simulink model "Chess_method_sowing_4_article"  (R2018b)
settings: Solver=FixedStepAuto  StartTime=0.0  StopTime=inf  FixedStep=0.01  MaxStep=0.01  MinStep=0.001  RelTol=1e-3  AbsTol=1e-3  EnableMultiTasking=on
libraries: fl_lib x6, nesl_utility x5, elec_lib x1
settings Model: Creator=Admin  LastModifiedBy=Admin
settings SolverCC: AutoInsertRateTranBlk=on  InsertRTBMode=Always

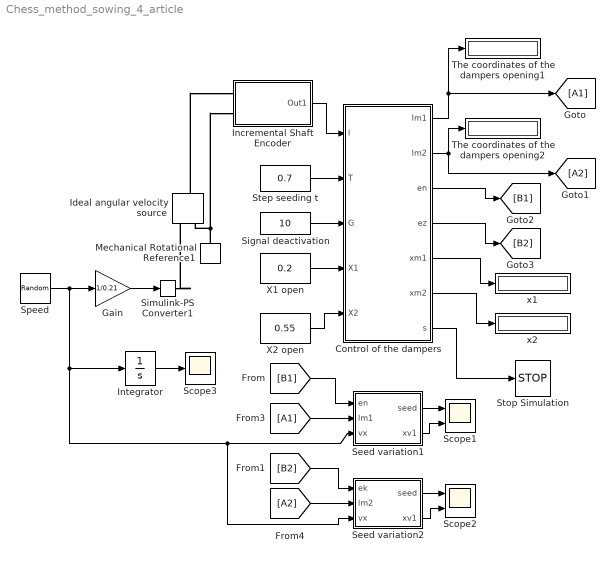
== system Chess_method_sowing_4_article ==
  Control of the dampers : MATLAB Function  TreatAsAtomicUnit=on
  Gain : Gain  Gain=1/0.21
  Ideal angular velocity source : fl_lib/Mechanical/Mechanical Sources/Ideal Angular Velocity Source
  Incremental Shaft Encoder : Subsystem
  Integrator : Integrator
  Mechanical Rotational Reference1 : fl_lib/Mechanical/Rotational Elements/Mechanical Rotational Reference
  Scope1 : Scope  NumInputPorts=2
  Scope2 : Scope  NumInputPorts=2
  Scope3 : Scope
  Seed variation1 : Subsystem
  Seed variation2 : Subsystem
  Signal deactivation : Constant  Value=10
  Simulink-PS Converter1 : nesl_utility/Simulink-PS Converter  PhysicalDomain=network_engine_domain  SubClassName=ps_input  LeftPortType=input  RightPortType=output  PseudoPeriodic=off  Frequencies=[]  NoiseDistribution=none  NoiseParameters=[]  Unit=rad/s  AffineConversion=off  FilteringAndDerivatives=provide  SimscapeFilterOrder=1  InputFilterTimeConstant=0.001  UdotUserProvided=0
  Speed : RandomNumber  Mean=2.5  Variance=0.1  SampleTime=0.1
  Step seeding t : Constant  Value=0.7
  Stop Simulation : Stop
  The coordinates of the dampers opening1 : Display
      settings: Format=bank
  The coordinates of the dampers opening2 : Display
      settings: Format=bank
  X1 open : Constant  Value=0.2  VectorParams1D=off
  X2 open : Constant  Value=0.55  VectorParams1D=off
  x1 : Display
      settings: Format=bank
  x2 : Display
      settings: Format=bank
  wires:
  Step seeding t/1 -> Control of the dampers/2(T)
  Control of the dampers/7(s) -> Stop Simulation/1
  Signal deactivation/1 -> Control of the dampers/3(G)
  X2 open/1 -> Control of the dampers/5(X2)
  Control of the dampers/6(xm2) -> x2/1
  Control of the dampers/5(xm1) -> x1/1
  X1 open/1 -> Control of the dampers/4(X1)
  Seed variation1/1(seed) -> Scope1/1
  Integrator/1 -> Scope3/1
  Speed/1 -> Seed variation1/3(vx), Seed variation2/3(vx), Integrator/1, Gain/1
  Seed variation1/2(xv1) -> Scope1/2
  [A1] -> Seed variation1/2(lm1)
  [A2] -> Seed variation2/2(lm2)
  Seed variation2/1(seed) -> Scope2/1
  Control of the dampers/2(lm2) -> The coordinates of the dampers opening2/1, [A2]
  Control of the dampers/1(lm1) -> [A1], The coordinates of the dampers opening1/1
  Seed variation2/2(xv1) -> Scope2/2
  Control of the dampers/3(en) -> [B1]
  Control of the dampers/4(ez) -> [B2]
  [B1] -> Seed variation1/1(en)
  [B2] -> Seed variation2/1(ek)
  Gain/1 -> Simulink-PS Converter1/1
  Incremental Shaft Encoder/1(Out1) -> Control of the dampers/1(l)
  connections:
  Simulink-PS Converter1/RConn1 -- Ideal angular velocity source/RConn1
  Mechanical Rotational Reference1/LConn1 -- Incremental Shaft Encoder/LConn2 -- Ideal angular velocity source/RConn2
  Ideal angular velocity source/LConn1 -- Incremental Shaft Encoder/LConn1

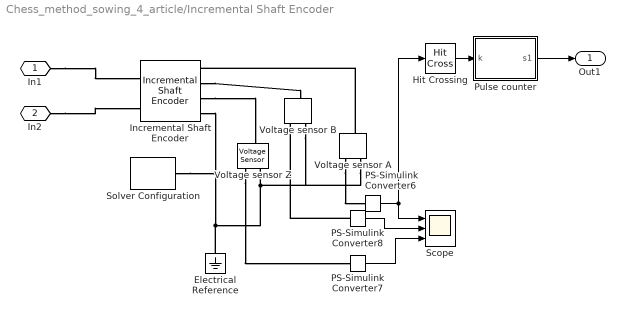
== system Chess_method_sowing_4_article/Incremental Shaft Encoder ==
  Electrical Reference : fl_lib/Electrical/Electrical Elements/Electrical Reference
  Hit Crossing : HitCross  HitCrossingOffset=0.6  HitCrossingDirection=rising
  Incremental Shaft Encoder : elec_lib/Sensors/Incremental Shaft Encoder  NPulse=852  Vm=1 V  angle0=0 rad
      settings: SourceProductName=Simscape Electronics  SourceProductBaseCode=SN
  PS-Simulink Converter6 : nesl_utility/PS-Simulink Converter  PhysicalDomain=network_engine_domain  SubClassName=ps_output  LeftPortType=input  RightPortType=output  PseudoPeriodic=off  Frequencies=[]  Unit=1  AffineConversion=off
  PS-Simulink Converter7 : nesl_utility/PS-Simulink Converter  PhysicalDomain=network_engine_domain  SubClassName=ps_output  LeftPortType=input  RightPortType=output  PseudoPeriodic=off  Frequencies=[]  Unit=1  AffineConversion=off
  PS-Simulink Converter8 : nesl_utility/PS-Simulink Converter  PhysicalDomain=network_engine_domain  SubClassName=ps_output  LeftPortType=input  RightPortType=output  PseudoPeriodic=off  Frequencies=[]  Unit=1  AffineConversion=off
  Pulse counter : MATLAB Function  TreatAsAtomicUnit=on
  Scope : Scope  NumInputPorts=3
  Solver Configuration : nesl_utility/Solver Configuration  PhysicalDomain=network_engine_domain  SubClassName=solver  LeftPortType=input  RightPortType=generic  Tones=[]  Harmonics=[]  SimulateNoise=off  Profile=off  UseLocalSampling=off  EnableSwitchedLinearOptims=on  FrequencyDomain=off  UseCCode=off  RelTol=0.001  AbsTol=1e-06  MinStep=1e-09  ToWorkspace=off  RevertToSquareIcSolve=off  NumHomotopyIterations=100  PhasorMode=off  PhasorModeNumHarmonics=1  DoDC=off  ResidualTolerance=1e-09  UseLocalSolver=off  LocalSolverChoice=NE_BACKWARD_EULER_ADVANCER  LocalSolverSampleTime=0.001  DoFixedCost=off  MaxNonlinIter=3  MaxModeIter=2  LinearAlgebra=auto  EquationFormulation=NE_TIME_EF  DelaysMemoryBudget=1024  AutomaticFiltering=on  FilteringTimeConstant=0.001  PartitionStorageMethod=AS_NEEDED  PartitionMemoryBudget=1024
  Voltage sensor A : fl_lib/Electrical/Electrical Sensors/Voltage Sensor
  Voltage sensor B : fl_lib/Electrical/Electrical Sensors/Voltage Sensor
  Voltage sensor Z : fl_lib/Electrical/Electrical Sensors/Voltage Sensor
  In1 : PMIOPort  Side=Left
  In2 : PMIOPort  Port=2  Side=Left
  Out1 : Outport
  wires:
  PS-Simulink Converter6/1 -> Scope/1, Hit Crossing/1
  Hit Crossing/1 -> Pulse counter/1("k ")
  PS-Simulink Converter8/1 -> Scope/2
  PS-Simulink Converter7/1 -> Scope/3
  Pulse counter/1(s1) -> Out1/1
  connections:
  Solver Configuration/RConn1 -- Incremental Shaft Encoder/RConn4 -- Electrical Reference/LConn1 -- Voltage sensor A/RConn2 -- Voltage sensor B/RConn2 -- Voltage sensor Z/RConn2
  Incremental Shaft Encoder/RConn3 -- Voltage sensor Z/LConn1
  Incremental Shaft Encoder/RConn2 -- Voltage sensor B/LConn1
  In2/RConn1 -- Incremental Shaft Encoder/LConn2
  Voltage sensor Z/RConn1 -- PS-Simulink Converter7/LConn1
  Voltage sensor A/LConn1 -- Incremental Shaft Encoder/RConn1
  Voltage sensor A/RConn1 -- PS-Simulink Converter6/LConn1
  PS-Simulink Converter8/LConn1 -- Voltage sensor B/RConn1
  In1/RConn1 -- Incremental Shaft Encoder/LConn1

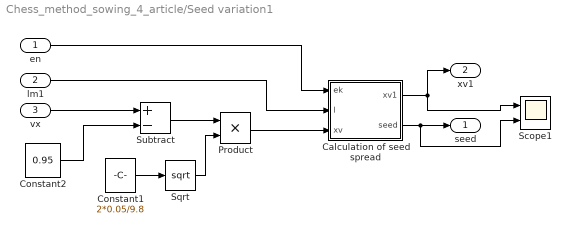
== system Chess_method_sowing_4_article/Seed variation1 ==
  en : Inport
  lm1 : Inport  Port=2
  vx : Inport  Port=3
  Calculation of seed spread : MATLAB Function  TreatAsAtomicUnit=on
  Constant1 : Constant  Value=2*0.05/9.8  VectorParams1D=off
  Constant2 : Constant  Value=0.95  VectorParams1D=off
  Product : Product
  Scope1 : Scope  NumInputPorts=2
  Sqrt : Sqrt  SaturateOnIntegerOverflow=on
  Subtract : Sum  Inputs=+-
  seed : Outport
  xv1 : Outport  Port=2
  wires:
  Calculation of seed spread/1(xv1) -> Scope1/1, xv1/1
  Calculation of seed spread/2(seed) -> Scope1/2, seed/1
  Sqrt/1 -> Product/2
  Constant2/1 -> Subtract/2
  vx/1 -> Subtract/1
  Subtract/1 -> Product/1
  lm1/1 -> Calculation of seed spread/2(l)
  Constant1/1 -> Sqrt/1
  en/1 -> Calculation of seed spread/1(ek)
  Product/1 -> Calculation of seed spread/3(xv)

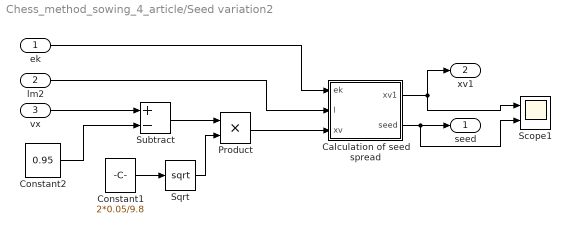
== system Chess_method_sowing_4_article/Seed variation2 ==
  ek : Inport
  lm2 : Inport  Port=2
  vx : Inport  Port=3
  Calculation of seed spread : MATLAB Function  TreatAsAtomicUnit=on
  Constant1 : Constant  Value=2*0.05/9.8  VectorParams1D=off
  Constant2 : Constant  Value=0.95  VectorParams1D=off
  Product : Product
  Scope1 : Scope  NumInputPorts=2
  Sqrt : Sqrt  SaturateOnIntegerOverflow=on
  Subtract : Sum  Inputs=+-
  seed : Outport
  xv1 : Outport  Port=2
  wires:
  Calculation of seed spread/1(xv1) -> Scope1/1, xv1/1
  Calculation of seed spread/2(seed) -> Scope1/2, seed/1
  Sqrt/1 -> Product/2
  Constant2/1 -> Subtract/2
  vx/1 -> Subtract/1
  Subtract/1 -> Product/1
  lm2/1 -> Calculation of seed spread/2(l)
  Constant1/1 -> Sqrt/1
  ek/1 -> Calculation of seed spread/1(ek)
  Product/1 -> Calculation of seed spread/3(xv)

== matlab function Chess_method_sowing_4_article/Seed variation2/Calculation of seed spread ==
  settings: updateMethod=DISCRETE
  data: ek input; xv1 output; l input; seed output; xv input
function [xv1,seed] = fcn(ek,l,xv)
seed=0;

persistent vx
if isempty(vx)  
    vx = 0;
end


persistent k
if isempty(k)  
    k = 1;
end

persistent j
if isempty(j)  
    j = 0;
end

persistent m
if isempty(m)  
    m = 0;
end

persistent n1
if isempty(n1)  
    n1 = 0;
end


if ek==1
    m=l+xv;
    k=k+1;
    vx=xv;
end

if l>=m & l~=0 & k>j
    seed=1;
    n1=n1+1;
    j=j+1;
end

xv1=vx;
% seed;
n=n1;

== matlab function Chess_method_sowing_4_article/Incremental Shaft Encoder/Pulse counter ==
  settings: updateMethod=DISCRETE
  data: k input; s1 output
function s1  = fcn(k)

persistent s
if isempty(s)  
    s = 0;
end 

persistent n
if isempty(n)  
    n = 0;
end

if k>0
    s=s+1;
    n=s*2*pi*0.21/213;
    k;
   
else
    n
end

y=n
s1=s

== matlab function Chess_method_sowing_4_article/Seed variation1/Calculation of seed spread ==
  settings: updateMethod=DISCRETE
  data: ek input; xv1 output; l input; seed output; xv input
function [xv1,seed] = fcn(ek,l,xv)
seed=0;

persistent vx
if isempty(vx)  
    vx = 0;
end


persistent k
if isempty(k)  
    k = 1;
end

persistent j
if isempty(j)  
    j = 0;
end

persistent m
if isempty(m)  
    m = 0;
end

persistent n1
if isempty(n1)  
    n1 = 0;
end


if ek==1
    m=l+xv;
    k=k+1;
    vx=xv;
end

if l>=m & l~=0 & k>j
    seed=1;
    n1=n1+1;
    j=j+1;
end

xv1=vx;
% seed;
n=n1;

== matlab function Chess_method_sowing_4_article/Control of the dampers ==
  settings: updateMethod=DISCRETE
  data: l input; lm1 output; T input; lm2 output; en output; ez output; xm1 output; xm2 output; s output; G input; X1 input; X2 input
function [lm1, lm2, en, ez, xm1, xm2, s]= fcn(l, T, G, X1,X2)

s=0; %инициализация переменной для остановки программы 
     % в см симуляция выключения 
     %следящего устройства по сигналу спутника
en=0;   % моделирование сигнала октр. кл. нечетных секций        
ez=0;   % моделирование сигнала октр. кл. четных секций            

% определение переводного коэффициента kf (расстояние за 1 сигнал энкодера)
kf=2*pi*0.21/852; 

% перевод из метров в количество сигналов 
t=round(T/kf); %шаг посева
g=round(G/kf);  %расстояние деактивации энкодера

% перевод сигналов, поступающих из энкодера в метры
lm=l*kf;

% инициализация входных переменных
% локальные персистентные переменные
persistent nn  % кол-во откр. клапан. нечетных секций за один проход
persistent nz  % кол-во откр. клапан. четных секций за один проход
persistent ln  % расстояние на котором сработали нечетные клапаны
persistent lz  % расстояние на котором сработали четные клапаны
persistent xn  % расстояние отк. клап. в начале 1 и последующих проходов
persistent xz  % расстояние отк. клап. в начале 1 и последующих проходов

if isempty(nn)  
    nn = 0;
end

if isempty(nz)
    nz = 0;
end

if isempty(ln)
    ln = 0;
end

if isempty(lz)
    lz = 0;
end

if isempty(xn)
    xn = round(X1/kf); %количество сигналов с энкодера;
end

if isempty(xz)
    xz = round(X2/kf); %количество сигналов с энкодера;
end

% Запуск работы эл. клапанов.
if l==xz
   ln=l;
   lm1=ln*kf;
   en=1;  % откр. электроклапанов нечетных секций
   nn=nn+1; % кол-во отк. электроклапанов нечетных секций

elseif l==xn
        lz=l;
        lm2=lz*kf;
        ez=1;  % откр. электроклапанов четных секций
        nz=nz+1; % кол-во отк. электроклапанов четных секций

%сравнение текущей позиции сеялки с шагом посева
elseif l-ln == t 
            ln=l;
            lm1=ln*kf;
            en=1;  % откр. электроклапанов нечетных секций
            nn=nn+1; % кол-во отк. электроклапанов нечетных секций

elseif  l-ln == round((T/kf)/2) & ln~=0
                lz=l;
                lm2=lz*kf;
                ez=1;  % откр. электроклапанов нечетных секций
                nz=nz+1; % кол-во отк. электроклапанов нечетных секций
end

% симуляция выключения измерительного устройства
if l >= g  
    xn= l-ln;% запись расстояния последнего срабатывния заслонок на проходе.
    xm1=xn*kf;
    xz= l-lz; % запись расстояния последнего срабатывания заслонок на проходе.
    xm2=xz*kf;
    s=1; % отправка сигнала на блок STOP
end

% Вывод показателей работы и сигналов симулинк:
n1=nn;
n2=nz;
lm1=ln*kf;
lm2=lz*kf;
xm1=xn*kf;
xm2=xz*kf;
